simulink model "globalReroute_fsm"  (R2022a)
settings: Solver=VariableStepAuto  StartTime=0.0  StopTime=10.0  RelTol=1e-3
settings Model: Creator=Nate  LastModifiedBy=Antonio Alonso
settings DebuggingCC: UnconnectedInputMsg=warning  UnconnectedOutputMsg=warning  UnconnectedLineMsg=warning
settings RTWCC: DLArmComputeVersion=19.05

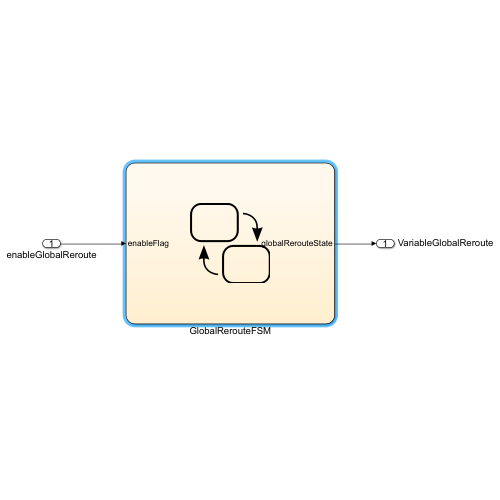
[thumbnail: Simulink's stored preview of the top-level diagram]
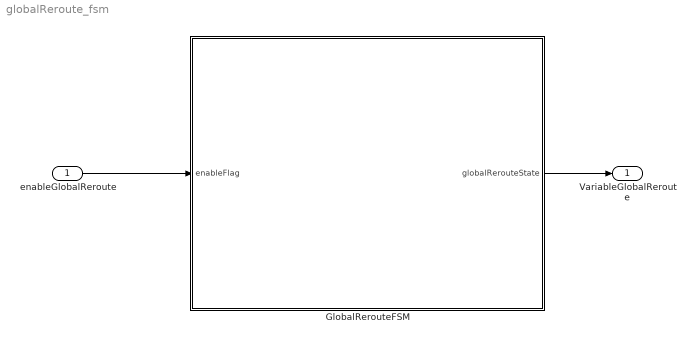
== system globalReroute_fsm ==
  enableGlobalReroute : Inport
  GlobalRerouteFSM : Stateflow chart  TreatAsAtomicUnit=on
  VariableGlobalReroute : Outport
  wires:
  GlobalRerouteFSM/1(globalRerouteState) -> VariableGlobalReroute/1
  enableGlobalReroute/1 -> GlobalRerouteFSM/1(enableFlag)

== stateflow chart globalReroute_fsm/GlobalRerouteFSM ==
  state wait_for_globalReroute_enable
    en:  globalRerouteState = 0;
  state waitToStop
    en:  globalRerouteState = 1;
    du: waitStop()
  state signalPathPlanning
    en:  globalRerouteState = 2
    ex: VariablePathPlan = 1;
  (default) -> wait_for_globalReroute_enable
  wait_for_globalReroute_enable -> wait_for_globalReroute_enable [order 2]
  signalPathPlanning -> wait_for_globalReroute_enable
  waitToStop -> wait_for_globalReroute_enable [order 2] : [VariableGlobalEnable ==false]
  wait_for_globalReroute_enable -> waitToStop [order 1] : [VariableGlobalReroute == true]
  waitToStop -> waitToStop [order 3]
  waitToStop -> signalPathPlanning [order 1] : [vCar == 0]
  data: ActiveObjectList data_store_memory; SpeedChangeEnable data_store_memory; VariableStopEnable data_store_memory; SubMachineRunning data_store_memory; curObstacle local; globalRerouteState output; enableFlag input
